simulink model "sim_topic2"  (R2023b)
settings: Solver=VariableStepAuto  StartTime=0.0  StopTime=N  RelTol=1e-3
undefined symbols (not defined in the file): Ad, Bd, Cd, Dd, T, xd0
settings Model: Creator=user  LastModifiedBy=user

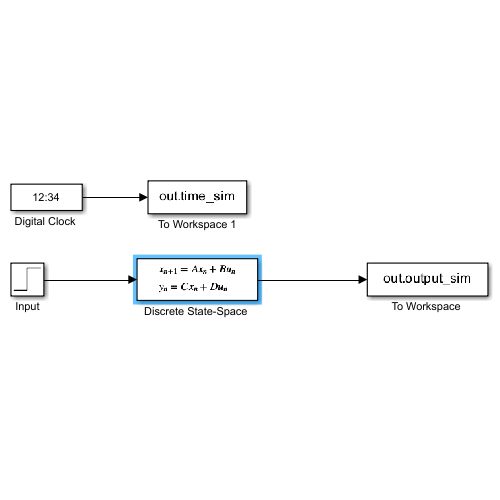
[thumbnail: Simulink's stored preview of the top-level diagram]
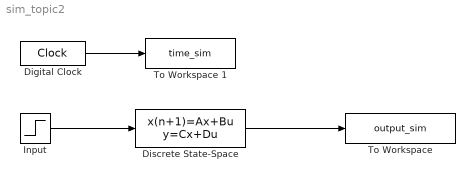
== system sim_topic2 ==
  "Digital Clock " : DigitalClock  SampleTime=T
  "Discrete State-Space " : DiscreteStateSpace  A=Ad  B=Bd  C=Cd  D=Dd  InitialCondition=xd0  SampleTime=T
  Input : Step  Time=0  SampleTime=T
  "To Workspace " : ToWorkspace  VariableName=output_sim  SampleTime=-1
  To Workspace 1 : ToWorkspace  VariableName=time_sim  SampleTime=-1
  wires:
  "Digital Clock "/1 -> To Workspace 1/1
  Input/1 -> "Discrete State-Space "/1
  "Discrete State-Space "/1 -> "To Workspace "/1
